simulink library "constYZTvarX_cl"  (R2022a)
settings: Solver=VariableStepAuto  StartTime=0.0  StopTime=10.0  RelTol=1e-3
undefined symbols (not defined in the file): amp, freq
settings Model: Creator=mcobb  LastModifiedBy=lhill8
settings SolverCC: AlgebraicLoopSolver=TrustRegion
settings DebuggingCC: UnconnectedInputMsg=warning  UnconnectedOutputMsg=warning  UnconnectedLineMsg=warning  SFMachineParentedDataDiag=warning  ArithmeticOperatorsInVariantConditions=warning
settings SFSimCC: CustomCodeUndefinedFunction=UseInterfaceOnly

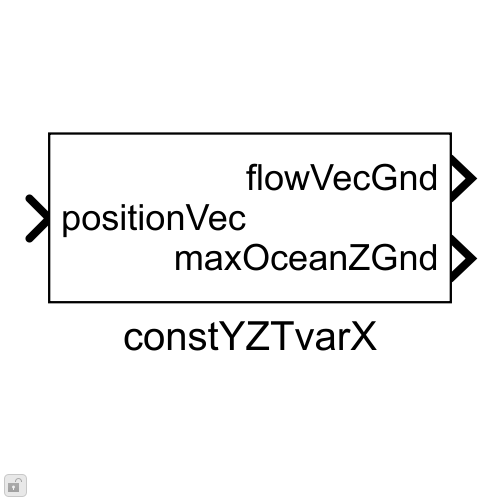
[thumbnail: Simulink's stored preview of the top-level diagram]
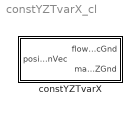
== system constYZTvarX_cl ==
  constYZTvarX : Subsystem  mask{constXYZT=0}
      mask prompts: constXYZT "env.constXYZT Object"

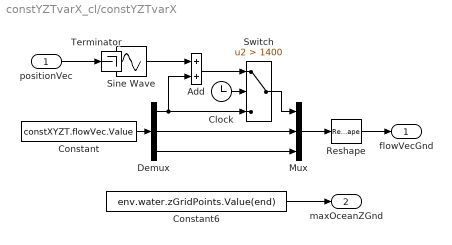
== system constYZTvarX_cl/constYZTvarX ==
  positionVec : Inport
  Add : Sum
  Clock : Clock
  Constant : Constant  Value=constXYZT.flowVec.Value
  Constant6 : Constant  Value=env.water.zGridPoints.Value(end)
  Demux : Demux  Outputs=3
  Mux : Mux  Inputs=3
  Reshape : Reshape  OutputDimensionality=Column vector (2-D)
  Sine Wave : Sin  Amplitude=amp  Frequency=freq  SampleTime=0
  Switch : Switch  Criteria=u2 > Threshold  Threshold=1400  SaturateOnIntegerOverflow=off  InputSameDT=off
  Terminator : Terminator
  flowVecGnd : Outport  VectorParamsAs1DForOutWhenUnconnected=off
  maxOceanZGnd : Outport  Port=2  VectorParamsAs1DForOutWhenUnconnected=off
  wires:
  positionVec/1 -> Terminator/1
  Reshape/1 -> flowVecGnd/1
  Constant6/1 -> maxOceanZGnd/1
  Constant/1 -> Demux/1
  Mux/1 -> Reshape/1
  Demux/2 -> Mux/2
  Demux/3 -> Mux/3
  Switch/1 -> Mux/1
  Clock/1 -> Switch/2
  Demux/1 -> Add/2, Switch/3
  Sine Wave/1 -> Add/1
  Add/1 -> Switch/1
